simulink model "linearpll"  (Simulink 8.4)
settings: Solver=ode45  StartTime=0.0  StopTime=100e-6  RelTol=1e-3
libraries: commsynccomp2 x1, dsparch4 x1
settings Model: Creator=Edwin Pasterkamp  LastModifiedBy=Mohamed Elreedy
settings OptimizationCC: InitFltsAndDblsToZero=on
settings DebuggingCC: SaveWithParameterizedLinksMsg=none  SignalResolutionControl=TryResolveAllWithWarning
settings GRTTargetCC: TargetFcnLib=ansi_tfl_tmw.mat

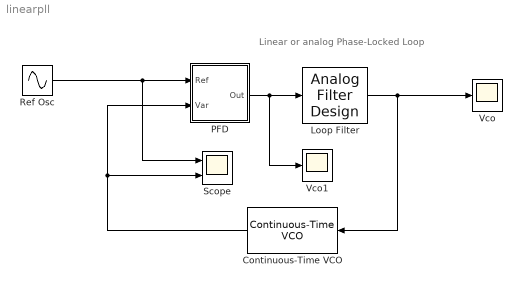
== system linearpll ==
  note: Linear or analog Phase-Locked Loop
  Continuous-Time VCO : commsynccomp2/Continuous-Time VCO  Ac=1  Fc=1e6  Kc=1e5  Ph=0
  Loop Filter : dsparch4/Analog Filter Design  method=Butterworth  filttype=Lowpass  N=7  Wlo=1e6*2*pi  Whi=80  Rp=1  Rs=180
  PFD : Subsystem
  Ref Osc : Sin  Frequency=2*pi*(1e6)  SampleTime=0
      settings: AttributesFormatString=%<Frequency> (rad/s)
  Scope : Scope  NumInputPorts=2
      settings: TimeRange=0.0001  YMin=-1.5~-1.5  YMax=1.5~1.5  SaveName=log_linearpll  SampleInput=on  SampleTime=1e-8
  Vco : Scope
      settings: TimeRange=0.0001  YMin=-1  YMax=1
  Vco1 : Scope
      settings: TimeRange=0.0001  YMin=-1  YMax=1
  wires:
  Ref Osc/1 -> Scope/1, PFD/1(Ref)
  PFD/1(Out) -> Vco1/1, Loop Filter/1
  Loop Filter/1 -> Vco/1, Continuous-Time VCO/1
  Continuous-Time VCO/1 -> Scope/2, PFD/2(Var)

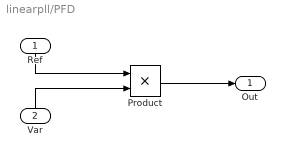
== system linearpll/PFD ==
  Ref : Inport
  Var : Inport  Port=2
  Product : Product  RndMeth=Zero
  Out : Outport
  wires:
  Ref/1 -> Product/1
  Var/1 -> Product/2
  Product/1 -> Out/1
